simulink model "ProgramCounter"  (R2024b)
settings: Solver=FixedStepAuto  StartTime=0.0  StopTime=10  FixedStep=1e-6  RelTol=1e-3
libraries: simulink_extras x13
settings Model: PacingRate=0.002500  Creator=Erys  LastModifiedBy=Erys
settings SolverCC: AllowMultiTaskInputOutput=on

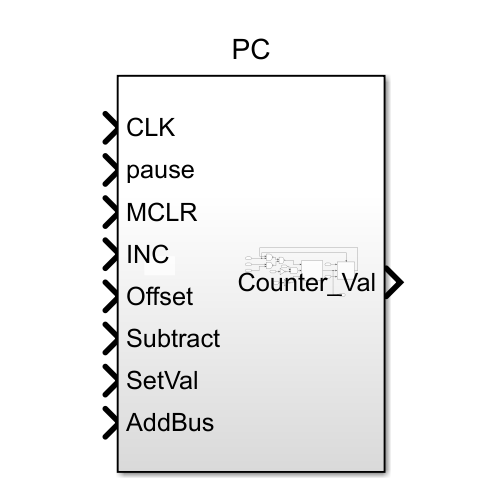
[thumbnail: Simulink's stored preview of the top-level diagram]
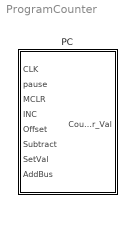
== system ProgramCounter ==
  PC : Subsystem

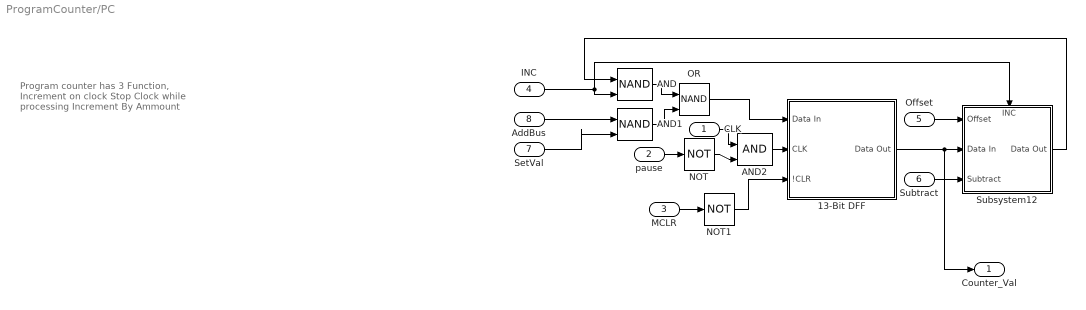
== system ProgramCounter/PC ==
  note: Program counter has 3 Function,
      |
      | Increment on clock
      | Stop Clock while processing
      | Increment By Ammount
  CLK : Inport
  pause : Inport  Port=2
  MCLR : Inport  Port=3
  INC : Inport  Port=4
  Offset : Inport  Port=5
  Subtract : Inport  Port=6
  SetVal : Inport  Port=7
  AddBus : Inport  Port=8
  "13-Bit DFF " : Subsystem
  AND : Logic  Operator=NAND  IconShape=distinctive  AllPortsSameDT=off  OutDataTypeStr=boolean
  AND1 : Logic  Operator=NAND  IconShape=distinctive  AllPortsSameDT=off  OutDataTypeStr=boolean
  AND2 : Logic  IconShape=distinctive  AllPortsSameDT=off  OutDataTypeStr=boolean
  NOT : Logic  Operator=NOT  IconShape=distinctive  AllPortsSameDT=off  OutDataTypeStr=boolean
  NOT1 : Logic  Operator=NOT  IconShape=distinctive  AllPortsSameDT=off  OutDataTypeStr=boolean
  OR : Logic  Operator=NAND  IconShape=distinctive  AllPortsSameDT=off  OutDataTypeStr=boolean
  Subsystem12 : Subsystem
      settings: PortSchema="{\"entries\":[{\"content\":{\"sides\":[{\"content\":{\"connectorIds\":[\"In1\",\"In2\",\"In3\"]},\"type\":\"ConnectorPlacement.EquallySpacedRectSide\",\"uuid\":\"739cec16-4094-4955-9615-f23c4a15ab23\"},{\"content\":{\"connectorIds\":[\"Out1\"],\"side\":\"RIGHT\"},\"type\":\"ConnectorPlacement.EquallySpacedRectSide\",\"uuid\":\"36202d39-d5af-435f-89aa-f53363edb9fe\"},{\"content\":{\"connectorIds\":[\"In4\"],\"side\":\"TOP\"},\"type\":\"ConnectorPlacement.EquallySpacedRectSide\",\"uuid\":\"08216fe9-0399-4cf5-9d97-18b54c3decd6\"}]},\"type\":\"ConnectorPlacement.EquallySpacedConnector\",\"uuid\":\"ce037f61-d800-42dc-bcb7-acda0bd23fde\"}],\"packageUris\":[\"http://schema.mathworks.com/mf0/Connector/R2020b\"],\"version\":\"1.0\"}"
  Counter_Val : Outport
  wires:
  CLK/1 -> AND2/1
  MCLR/1 -> NOT1/1
  "13-Bit DFF "/1(Data Out) -> Counter_Val/1, Subsystem12/2(Data In)
  Subsystem12/1(Data Out) -> AND/1
  AND/1 -> OR/1
  AND1/1 -> OR/2
  OR/1 -> "13-Bit DFF "/1(Data In)
  Offset/1 -> Subsystem12/1(Offset)
  INC/1 -> AND/2, Subsystem12/4(INC)
  Subtract/1 -> Subsystem12/3(Subtract)
  SetVal/1 -> AND1/2
  AddBus/1 -> AND1/1
  NOT/1 -> AND2/2
  pause/1 -> NOT/1
  NOT1/1 -> "13-Bit DFF "/3(!CLR)
  AND2/1 -> "13-Bit DFF "/2(CLK)

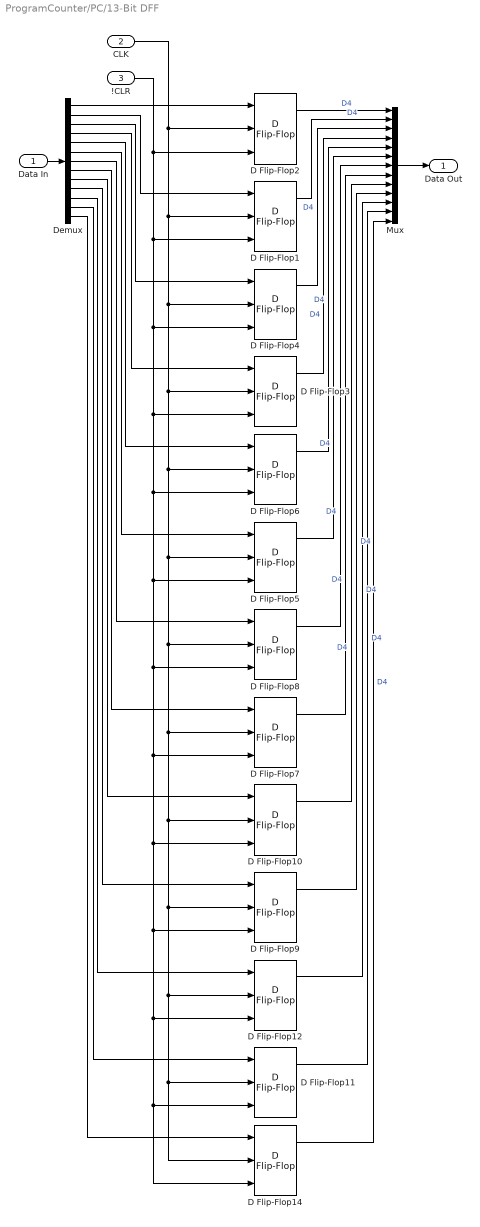
== system ProgramCounter/PC/13-Bit DFF  ==
  Data In : Inport
  CLK : Inport  Port=2
  !CLR : Inport  Port=3
  D Flip-Flop{1..12,14} (13 alike) : simulink_extras/Flip Flops/D Flip-Flop
  Demux : Demux  Outputs=13
  Mux : Mux  Inputs=13
  Data Out : Outport
  wires:
  Data In/1 -> Demux/1
  Mux/1 -> Data Out/1
  !CLR/1 -> D Flip-Flop4/3, D Flip-Flop3/3, D Flip-Flop6/3, D Flip-Flop8/3, D Flip-Flop12/3, D Flip-Flop11/3, D Flip-Flop14/3, D Flip-Flop9/3, D Flip-Flop10/3, D Flip-Flop7/3, D Flip-Flop5/3, D Flip-Flop1/3, D Flip-Flop2/3
  CLK/1 -> D Flip-Flop1/2, D Flip-Flop6/2, D Flip-Flop5/2, D Flip-Flop8/2, D Flip-Flop9/2, D Flip-Flop14/2, D Flip-Flop11/2, D Flip-Flop12/2, D Flip-Flop10/2, D Flip-Flop7/2, D Flip-Flop3/2, D Flip-Flop4/2, D Flip-Flop2/2
  Demux/1 -> D Flip-Flop2/1
  Demux/2 -> D Flip-Flop1/1
  Demux/3 -> D Flip-Flop4/1
  Demux/4 -> D Flip-Flop3/1
  Demux/5 -> D Flip-Flop6/1
  Demux/6 -> D Flip-Flop5/1
  Demux/7 -> D Flip-Flop8/1
  Demux/8 -> D Flip-Flop7/1
  Demux/9 -> D Flip-Flop10/1
  Demux/10 -> D Flip-Flop9/1
  Demux/11 -> D Flip-Flop12/1
  Demux/12 -> D Flip-Flop11/1
  Demux/13 -> D Flip-Flop14/1
  D Flip-Flop2/1 -> Mux/1  "D4"
  D Flip-Flop1/1 -> Mux/2  "D4"
  D Flip-Flop4/1 -> Mux/3  "D4"
  D Flip-Flop3/1 -> Mux/4  "D4"
  D Flip-Flop6/1 -> Mux/5  "D4"
  D Flip-Flop5/1 -> Mux/6  "D4"
  D Flip-Flop8/1 -> Mux/7  "D4"
  D Flip-Flop7/1 -> Mux/8  "D4"
  D Flip-Flop10/1 -> Mux/9  "D4"
  D Flip-Flop9/1 -> Mux/10  "D4"
  D Flip-Flop12/1 -> Mux/11  "D4"
  D Flip-Flop11/1 -> Mux/12  "D4"
  D Flip-Flop14/1 -> Mux/13  "D4"

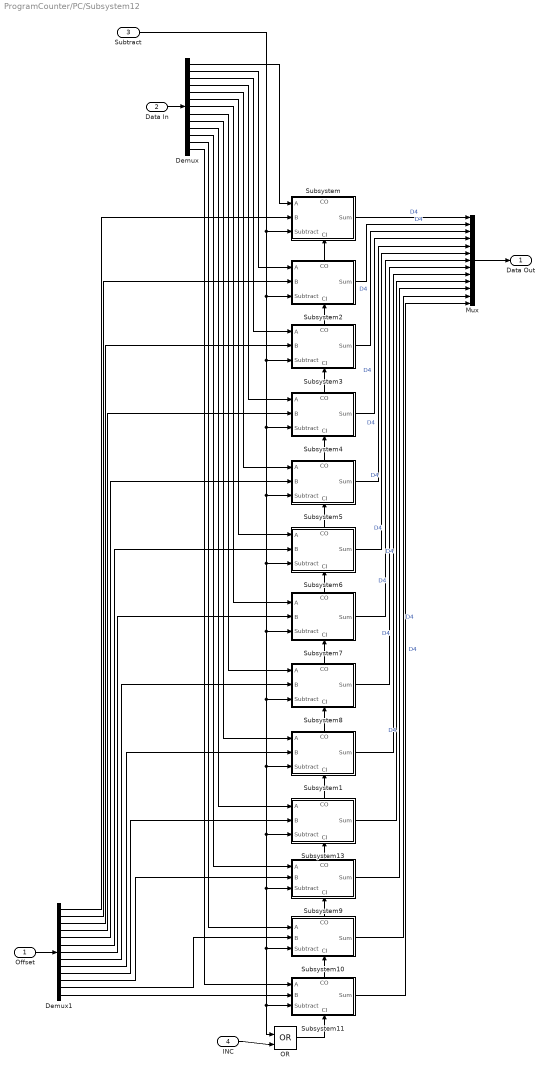
== system ProgramCounter/PC/Subsystem12 ==
  Offset : Inport
  Data In : Inport  Port=2
  Subtract : Inport  Port=3
  INC : Inport  Port=4
  Demux : Demux  Outputs=13
  Demux1 : Demux  Outputs=13
  Mux : Mux  Inputs=13
  OR : Logic  Operator=OR  IconShape=distinctive  AllPortsSameDT=off  OutDataTypeStr=boolean
  Subsystem : Subsystem
      settings: PortSchema="{\"entries\":[{\"content\":{\"sides\":[{\"content\":{\"connectorIds\":[\"In1\",\"In2\",\"In3\"]},\"type\":\"ConnectorPlacement.EquallySpacedRectSide\",\"uuid\":\"3b61df12-5278-441c-99ea-cd13bbe6a5f0\"},{\"content\":{\"connectorIds\":[\"Out1\"],\"side\":\"RIGHT\"},\"type\":\"ConnectorPlacement.EquallySpacedRectSide\",\"uuid\":\"d74b7cc5-7b27-4e0f-8d84-952eb44d2cfa\"},{\"content\":{\"connectorIds\":[\"Out2\"],\"side\":\"TOP\"},\"type\":\"ConnectorPlacement.EquallySpacedRectSide\",\"uuid\":\"99314f25-b6d9-4ea5-a032-83307ae4bc34\"},{\"content\":{\"connectorIds\":[\"In4\"],\"side\":\"BOTTOM\"},\"type\":\"ConnectorPlacement.EquallySpacedRectSide\",\"uuid\":\"c9c43d88-8d1b-4564-af22-30722c8258ba\"}]},\"type\":\"ConnectorPlacement.EquallySpacedConnector\",\"uuid\":\"25cc7102-d96a-4215-b1b2-f44cf7e448cb\"}],\"packageUris\":[\"http://schema.mathworks.com/mf0/Connector/R2020b\"],\"version\":\"1.0\"}"
  Subsystem1 : Subsystem
      settings: PortSchema="{\"entries\":[{\"content\":{\"sides\":[{\"content\":{\"connectorIds\":[\"In1\",\"In2\",\"In3\"]},\"type\":\"ConnectorPlacement.EquallySpacedRectSide\",\"uuid\":\"3b61df12-5278-441c-99ea-cd13bbe6a5f0\"},{\"content\":{\"connectorIds\":[\"Out1\"],\"side\":\"RIGHT\"},\"type\":\"ConnectorPlacement.EquallySpacedRectSide\",\"uuid\":\"d74b7cc5-7b27-4e0f-8d84-952eb44d2cfa\"},{\"content\":{\"connectorIds\":[\"Out2\"],\"side\":\"TOP\"},\"type\":\"ConnectorPlacement.EquallySpacedRectSide\",\"uuid\":\"99314f25-b6d9-4ea5-a032-83307ae4bc34\"},{\"content\":{\"connectorIds\":[\"In4\"],\"side\":\"BOTTOM\"},\"type\":\"ConnectorPlacement.EquallySpacedRectSide\",\"uuid\":\"c9c43d88-8d1b-4564-af22-30722c8258ba\"}]},\"type\":\"ConnectorPlacement.EquallySpacedConnector\",\"uuid\":\"25cc7102-d96a-4215-b1b2-f44cf7e448cb\"}],\"packageUris\":[\"http://schema.mathworks.com/mf0/Connector/R2020b\"],\"version\":\"1.0\"}"
  Subsystem10 : Subsystem
      settings: PortSchema="{\"entries\":[{\"content\":{\"sides\":[{\"content\":{\"connectorIds\":[\"In1\",\"In2\",\"In3\"]},\"type\":\"ConnectorPlacement.EquallySpacedRectSide\",\"uuid\":\"3b61df12-5278-441c-99ea-cd13bbe6a5f0\"},{\"content\":{\"connectorIds\":[\"Out1\"],\"side\":\"RIGHT\"},\"type\":\"ConnectorPlacement.EquallySpacedRectSide\",\"uuid\":\"d74b7cc5-7b27-4e0f-8d84-952eb44d2cfa\"},{\"content\":{\"connectorIds\":[\"Out2\"],\"side\":\"TOP\"},\"type\":\"ConnectorPlacement.EquallySpacedRectSide\",\"uuid\":\"99314f25-b6d9-4ea5-a032-83307ae4bc34\"},{\"content\":{\"connectorIds\":[\"In4\"],\"side\":\"BOTTOM\"},\"type\":\"ConnectorPlacement.EquallySpacedRectSide\",\"uuid\":\"c9c43d88-8d1b-4564-af22-30722c8258ba\"}]},\"type\":\"ConnectorPlacement.EquallySpacedConnector\",\"uuid\":\"25cc7102-d96a-4215-b1b2-f44cf7e448cb\"}],\"packageUris\":[\"http://schema.mathworks.com/mf0/Connector/R2020b\"],\"version\":\"1.0\"}"
  Subsystem11 : Subsystem
      settings: PortSchema="{\"entries\":[{\"content\":{\"sides\":[{\"content\":{\"connectorIds\":[\"In1\",\"In2\",\"In3\"]},\"type\":\"ConnectorPlacement.EquallySpacedRectSide\",\"uuid\":\"3b61df12-5278-441c-99ea-cd13bbe6a5f0\"},{\"content\":{\"connectorIds\":[\"Out1\"],\"side\":\"RIGHT\"},\"type\":\"ConnectorPlacement.EquallySpacedRectSide\",\"uuid\":\"d74b7cc5-7b27-4e0f-8d84-952eb44d2cfa\"},{\"content\":{\"connectorIds\":[\"Out2\"],\"side\":\"TOP\"},\"type\":\"ConnectorPlacement.EquallySpacedRectSide\",\"uuid\":\"99314f25-b6d9-4ea5-a032-83307ae4bc34\"},{\"content\":{\"connectorIds\":[\"In4\"],\"side\":\"BOTTOM\"},\"type\":\"ConnectorPlacement.EquallySpacedRectSide\",\"uuid\":\"c9c43d88-8d1b-4564-af22-30722c8258ba\"}]},\"type\":\"ConnectorPlacement.EquallySpacedConnector\",\"uuid\":\"25cc7102-d96a-4215-b1b2-f44cf7e448cb\"}],\"packageUris\":[\"http://schema.mathworks.com/mf0/Connector/R2020b\"],\"version\":\"1.0\"}"
  Subsystem13 : Subsystem
      settings: PortSchema="{\"entries\":[{\"content\":{\"sides\":[{\"content\":{\"connectorIds\":[\"In1\",\"In2\",\"In3\"]},\"type\":\"ConnectorPlacement.EquallySpacedRectSide\",\"uuid\":\"3b61df12-5278-441c-99ea-cd13bbe6a5f0\"},{\"content\":{\"connectorIds\":[\"Out1\"],\"side\":\"RIGHT\"},\"type\":\"ConnectorPlacement.EquallySpacedRectSide\",\"uuid\":\"d74b7cc5-7b27-4e0f-8d84-952eb44d2cfa\"},{\"content\":{\"connectorIds\":[\"Out2\"],\"side\":\"TOP\"},\"type\":\"ConnectorPlacement.EquallySpacedRectSide\",\"uuid\":\"99314f25-b6d9-4ea5-a032-83307ae4bc34\"},{\"content\":{\"connectorIds\":[\"In4\"],\"side\":\"BOTTOM\"},\"type\":\"ConnectorPlacement.EquallySpacedRectSide\",\"uuid\":\"c9c43d88-8d1b-4564-af22-30722c8258ba\"}]},\"type\":\"ConnectorPlacement.EquallySpacedConnector\",\"uuid\":\"25cc7102-d96a-4215-b1b2-f44cf7e448cb\"}],\"packageUris\":[\"http://schema.mathworks.com/mf0/Connector/R2020b\"],\"version\":\"1.0\"}"
  Subsystem2 : Subsystem
      settings: PortSchema="{\"entries\":[{\"content\":{\"sides\":[{\"content\":{\"connectorIds\":[\"In1\",\"In2\",\"In3\"]},\"type\":\"ConnectorPlacement.EquallySpacedRectSide\",\"uuid\":\"3b61df12-5278-441c-99ea-cd13bbe6a5f0\"},{\"content\":{\"connectorIds\":[\"Out1\"],\"side\":\"RIGHT\"},\"type\":\"ConnectorPlacement.EquallySpacedRectSide\",\"uuid\":\"d74b7cc5-7b27-4e0f-8d84-952eb44d2cfa\"},{\"content\":{\"connectorIds\":[\"Out2\"],\"side\":\"TOP\"},\"type\":\"ConnectorPlacement.EquallySpacedRectSide\",\"uuid\":\"99314f25-b6d9-4ea5-a032-83307ae4bc34\"},{\"content\":{\"connectorIds\":[\"In4\"],\"side\":\"BOTTOM\"},\"type\":\"ConnectorPlacement.EquallySpacedRectSide\",\"uuid\":\"c9c43d88-8d1b-4564-af22-30722c8258ba\"}]},\"type\":\"ConnectorPlacement.EquallySpacedConnector\",\"uuid\":\"25cc7102-d96a-4215-b1b2-f44cf7e448cb\"}],\"packageUris\":[\"http://schema.mathworks.com/mf0/Connector/R2020b\"],\"version\":\"1.0\"}"
  Subsystem3 : Subsystem
      settings: PortSchema="{\"entries\":[{\"content\":{\"sides\":[{\"content\":{\"connectorIds\":[\"In1\",\"In2\",\"In3\"]},\"type\":\"ConnectorPlacement.EquallySpacedRectSide\",\"uuid\":\"3b61df12-5278-441c-99ea-cd13bbe6a5f0\"},{\"content\":{\"connectorIds\":[\"Out1\"],\"side\":\"RIGHT\"},\"type\":\"ConnectorPlacement.EquallySpacedRectSide\",\"uuid\":\"d74b7cc5-7b27-4e0f-8d84-952eb44d2cfa\"},{\"content\":{\"connectorIds\":[\"Out2\"],\"side\":\"TOP\"},\"type\":\"ConnectorPlacement.EquallySpacedRectSide\",\"uuid\":\"99314f25-b6d9-4ea5-a032-83307ae4bc34\"},{\"content\":{\"connectorIds\":[\"In4\"],\"side\":\"BOTTOM\"},\"type\":\"ConnectorPlacement.EquallySpacedRectSide\",\"uuid\":\"c9c43d88-8d1b-4564-af22-30722c8258ba\"}]},\"type\":\"ConnectorPlacement.EquallySpacedConnector\",\"uuid\":\"25cc7102-d96a-4215-b1b2-f44cf7e448cb\"}],\"packageUris\":[\"http://schema.mathworks.com/mf0/Connector/R2020b\"],\"version\":\"1.0\"}"
  Subsystem4 : Subsystem
      settings: PortSchema="{\"entries\":[{\"content\":{\"sides\":[{\"content\":{\"connectorIds\":[\"In1\",\"In2\",\"In3\"]},\"type\":\"ConnectorPlacement.EquallySpacedRectSide\",\"uuid\":\"3b61df12-5278-441c-99ea-cd13bbe6a5f0\"},{\"content\":{\"connectorIds\":[\"Out1\"],\"side\":\"RIGHT\"},\"type\":\"ConnectorPlacement.EquallySpacedRectSide\",\"uuid\":\"d74b7cc5-7b27-4e0f-8d84-952eb44d2cfa\"},{\"content\":{\"connectorIds\":[\"Out2\"],\"side\":\"TOP\"},\"type\":\"ConnectorPlacement.EquallySpacedRectSide\",\"uuid\":\"99314f25-b6d9-4ea5-a032-83307ae4bc34\"},{\"content\":{\"connectorIds\":[\"In4\"],\"side\":\"BOTTOM\"},\"type\":\"ConnectorPlacement.EquallySpacedRectSide\",\"uuid\":\"c9c43d88-8d1b-4564-af22-30722c8258ba\"}]},\"type\":\"ConnectorPlacement.EquallySpacedConnector\",\"uuid\":\"25cc7102-d96a-4215-b1b2-f44cf7e448cb\"}],\"packageUris\":[\"http://schema.mathworks.com/mf0/Connector/R2020b\"],\"version\":\"1.0\"}"
  Subsystem5 : Subsystem
      settings: PortSchema="{\"entries\":[{\"content\":{\"sides\":[{\"content\":{\"connectorIds\":[\"In1\",\"In2\",\"In3\"]},\"type\":\"ConnectorPlacement.EquallySpacedRectSide\",\"uuid\":\"3b61df12-5278-441c-99ea-cd13bbe6a5f0\"},{\"content\":{\"connectorIds\":[\"Out1\"],\"side\":\"RIGHT\"},\"type\":\"ConnectorPlacement.EquallySpacedRectSide\",\"uuid\":\"d74b7cc5-7b27-4e0f-8d84-952eb44d2cfa\"},{\"content\":{\"connectorIds\":[\"Out2\"],\"side\":\"TOP\"},\"type\":\"ConnectorPlacement.EquallySpacedRectSide\",\"uuid\":\"99314f25-b6d9-4ea5-a032-83307ae4bc34\"},{\"content\":{\"connectorIds\":[\"In4\"],\"side\":\"BOTTOM\"},\"type\":\"ConnectorPlacement.EquallySpacedRectSide\",\"uuid\":\"c9c43d88-8d1b-4564-af22-30722c8258ba\"}]},\"type\":\"ConnectorPlacement.EquallySpacedConnector\",\"uuid\":\"25cc7102-d96a-4215-b1b2-f44cf7e448cb\"}],\"packageUris\":[\"http://schema.mathworks.com/mf0/Connector/R2020b\"],\"version\":\"1.0\"}"
  Subsystem6 : Subsystem
      settings: PortSchema="{\"entries\":[{\"content\":{\"sides\":[{\"content\":{\"connectorIds\":[\"In1\",\"In2\",\"In3\"]},\"type\":\"ConnectorPlacement.EquallySpacedRectSide\",\"uuid\":\"3b61df12-5278-441c-99ea-cd13bbe6a5f0\"},{\"content\":{\"connectorIds\":[\"Out1\"],\"side\":\"RIGHT\"},\"type\":\"ConnectorPlacement.EquallySpacedRectSide\",\"uuid\":\"d74b7cc5-7b27-4e0f-8d84-952eb44d2cfa\"},{\"content\":{\"connectorIds\":[\"Out2\"],\"side\":\"TOP\"},\"type\":\"ConnectorPlacement.EquallySpacedRectSide\",\"uuid\":\"99314f25-b6d9-4ea5-a032-83307ae4bc34\"},{\"content\":{\"connectorIds\":[\"In4\"],\"side\":\"BOTTOM\"},\"type\":\"ConnectorPlacement.EquallySpacedRectSide\",\"uuid\":\"c9c43d88-8d1b-4564-af22-30722c8258ba\"}]},\"type\":\"ConnectorPlacement.EquallySpacedConnector\",\"uuid\":\"25cc7102-d96a-4215-b1b2-f44cf7e448cb\"}],\"packageUris\":[\"http://schema.mathworks.com/mf0/Connector/R2020b\"],\"version\":\"1.0\"}"
  Subsystem7 : Subsystem
      settings: PortSchema="{\"entries\":[{\"content\":{\"sides\":[{\"content\":{\"connectorIds\":[\"In1\",\"In2\",\"In3\"]},\"type\":\"ConnectorPlacement.EquallySpacedRectSide\",\"uuid\":\"3b61df12-5278-441c-99ea-cd13bbe6a5f0\"},{\"content\":{\"connectorIds\":[\"Out1\"],\"side\":\"RIGHT\"},\"type\":\"ConnectorPlacement.EquallySpacedRectSide\",\"uuid\":\"d74b7cc5-7b27-4e0f-8d84-952eb44d2cfa\"},{\"content\":{\"connectorIds\":[\"Out2\"],\"side\":\"TOP\"},\"type\":\"ConnectorPlacement.EquallySpacedRectSide\",\"uuid\":\"99314f25-b6d9-4ea5-a032-83307ae4bc34\"},{\"content\":{\"connectorIds\":[\"In4\"],\"side\":\"BOTTOM\"},\"type\":\"ConnectorPlacement.EquallySpacedRectSide\",\"uuid\":\"c9c43d88-8d1b-4564-af22-30722c8258ba\"}]},\"type\":\"ConnectorPlacement.EquallySpacedConnector\",\"uuid\":\"25cc7102-d96a-4215-b1b2-f44cf7e448cb\"}],\"packageUris\":[\"http://schema.mathworks.com/mf0/Connector/R2020b\"],\"version\":\"1.0\"}"
  Subsystem8 : Subsystem
      settings: PortSchema="{\"entries\":[{\"content\":{\"sides\":[{\"content\":{\"connectorIds\":[\"In1\",\"In2\",\"In3\"]},\"type\":\"ConnectorPlacement.EquallySpacedRectSide\",\"uuid\":\"3b61df12-5278-441c-99ea-cd13bbe6a5f0\"},{\"content\":{\"connectorIds\":[\"Out1\"],\"side\":\"RIGHT\"},\"type\":\"ConnectorPlacement.EquallySpacedRectSide\",\"uuid\":\"d74b7cc5-7b27-4e0f-8d84-952eb44d2cfa\"},{\"content\":{\"connectorIds\":[\"Out2\"],\"side\":\"TOP\"},\"type\":\"ConnectorPlacement.EquallySpacedRectSide\",\"uuid\":\"99314f25-b6d9-4ea5-a032-83307ae4bc34\"},{\"content\":{\"connectorIds\":[\"In4\"],\"side\":\"BOTTOM\"},\"type\":\"ConnectorPlacement.EquallySpacedRectSide\",\"uuid\":\"c9c43d88-8d1b-4564-af22-30722c8258ba\"}]},\"type\":\"ConnectorPlacement.EquallySpacedConnector\",\"uuid\":\"25cc7102-d96a-4215-b1b2-f44cf7e448cb\"}],\"packageUris\":[\"http://schema.mathworks.com/mf0/Connector/R2020b\"],\"version\":\"1.0\"}"
  Subsystem9 : Subsystem
      settings: PortSchema="{\"entries\":[{\"content\":{\"sides\":[{\"content\":{\"connectorIds\":[\"In1\",\"In2\",\"In3\"]},\"type\":\"ConnectorPlacement.EquallySpacedRectSide\",\"uuid\":\"3b61df12-5278-441c-99ea-cd13bbe6a5f0\"},{\"content\":{\"connectorIds\":[\"Out1\"],\"side\":\"RIGHT\"},\"type\":\"ConnectorPlacement.EquallySpacedRectSide\",\"uuid\":\"d74b7cc5-7b27-4e0f-8d84-952eb44d2cfa\"},{\"content\":{\"connectorIds\":[\"Out2\"],\"side\":\"TOP\"},\"type\":\"ConnectorPlacement.EquallySpacedRectSide\",\"uuid\":\"99314f25-b6d9-4ea5-a032-83307ae4bc34\"},{\"content\":{\"connectorIds\":[\"In4\"],\"side\":\"BOTTOM\"},\"type\":\"ConnectorPlacement.EquallySpacedRectSide\",\"uuid\":\"c9c43d88-8d1b-4564-af22-30722c8258ba\"}]},\"type\":\"ConnectorPlacement.EquallySpacedConnector\",\"uuid\":\"25cc7102-d96a-4215-b1b2-f44cf7e448cb\"}],\"packageUris\":[\"http://schema.mathworks.com/mf0/Connector/R2020b\"],\"version\":\"1.0\"}"
  Data Out : Outport
  wires:
  Demux/2 -> Subsystem2/1(A)
  Subtract/1 -> Subsystem/3(Subtract), OR/1, Subsystem11/3(Subtract), Subsystem10/3(Subtract), Subsystem9/3(Subtract), Subsystem13/3(Subtract), Subsystem1/3(Subtract), Subsystem8/3(Subtract), Subsystem7/3(Subtract), Subsystem6/3(Subtract), Subsystem5/3(Subtract), Subsystem4/3(Subtract), Subsystem3/3(Subtract), Subsystem2/3(Subtract)
  Subsystem8/2(CO) -> Subsystem7/4(CI)
  Demux/10 -> Subsystem13/1(A)
  Subsystem10/2(CO) -> Subsystem9/4(CI)
  Demux/1 -> Subsystem/1(A)
  Subsystem11/2(CO) -> Subsystem10/4(CI)
  Demux/5 -> Subsystem5/1(A)
  Subsystem10/1(Sum) -> Mux/12  "D4"
  Demux/7 -> Subsystem7/1(A)
  Subsystem3/1(Sum) -> Mux/3  "D4"
  Subsystem6/1(Sum) -> Mux/6  "D4"
  Demux/13 -> Subsystem11/1(A)
  Subsystem5/2(CO) -> Subsystem4/4(CI)
  Demux1/11 -> Subsystem9/2(B)
  OR/1 -> Subsystem11/4(CI)
  Demux1/12 -> Subsystem10/2(B)
  Offset/1 -> Demux1/1
  Subsystem2/1(Sum) -> Mux/2  "D4"
  Demux1/9 -> Subsystem1/2(B)
  INC/1 -> OR/2
  Demux1/13 -> Subsystem11/2(B)
  Demux1/8 -> Subsystem8/2(B)
  Demux1/10 -> Subsystem13/2(B)
  Demux1/2 -> Subsystem2/2(B)
  Demux1/1 -> Subsystem/2(B)
  Demux1/6 -> Subsystem6/2(B)
  Subsystem/1(Sum) -> Mux/1  "D4"
  Demux1/3 -> Subsystem3/2(B)
  Demux1/7 -> Subsystem7/2(B)
  Demux1/4 -> Subsystem4/2(B)
  Subsystem4/2(CO) -> Subsystem3/4(CI)
  Subsystem7/1(Sum) -> Mux/7  "D4"
  Demux/6 -> Subsystem6/1(A)
  Subsystem6/2(CO) -> Subsystem5/4(CI)
  Demux1/5 -> Subsystem5/2(B)
  Subsystem7/2(CO) -> Subsystem6/4(CI)
  Subsystem3/2(CO) -> Subsystem2/4(CI)
  Subsystem5/1(Sum) -> Mux/5  "D4"
  Subsystem2/2(CO) -> Subsystem/4(CI)
  Subsystem1/1(Sum) -> Mux/9  "D4"
  Subsystem8/1(Sum) -> Mux/8  "D4"
  Subsystem11/1(Sum) -> Mux/13  "D4"
  Subsystem13/2(CO) -> Subsystem1/4(CI)
  Subsystem9/1(Sum) -> Mux/11  "D4"
  Subsystem1/2(CO) -> Subsystem8/4(CI)
  Demux/9 -> Subsystem1/1(A)
  Demux/11 -> Subsystem9/1(A)
  Mux/1 -> Data Out/1
  Subsystem9/2(CO) -> Subsystem13/4(CI)
  Subsystem13/1(Sum) -> Mux/10  "D4"
  Demux/8 -> Subsystem8/1(A)
  Demux/4 -> Subsystem4/1(A)
  Data In/1 -> Demux/1
  Subsystem4/1(Sum) -> Mux/4  "D4"
  Demux/3 -> Subsystem3/1(A)
  Demux/12 -> Subsystem10/1(A)

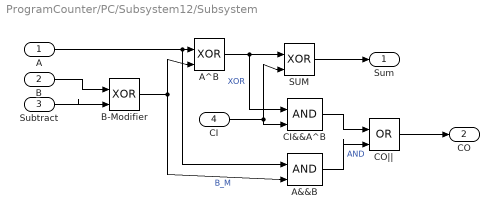
== system ProgramCounter/PC/Subsystem12/Subsystem ==
  A : Inport
  B : Inport  Port=2
  Subtract : Inport  Port=3
  CI : Inport  Port=4
  A&&B : Logic  IconShape=distinctive  AllPortsSameDT=off  OutDataTypeStr=boolean
  A^B : Logic  Operator=XOR  IconShape=distinctive  AllPortsSameDT=off  OutDataTypeStr=boolean
  B-Modifier : Logic  Operator=XOR  IconShape=distinctive  AllPortsSameDT=off  OutDataTypeStr=boolean
  CI&&A^B : Logic  IconShape=distinctive  AllPortsSameDT=off  OutDataTypeStr=boolean
  CO|| : Logic  Operator=OR  IconShape=distinctive  AllPortsSameDT=off  OutDataTypeStr=boolean
  SUM : Logic  Operator=XOR  IconShape=distinctive  AllPortsSameDT=off  OutDataTypeStr=boolean
  Sum : Outport
  CO : Outport  Port=2
  wires:
  B/1 -> B-Modifier/1
  Subtract/1 -> B-Modifier/2
  CI&&A^B/1 -> CO||/1
  A&&B/1 -> CO||/2  "AND"
  CO||/1 -> CO/1
  B-Modifier/1 -> A&&B/2, A^B/2  "B_M"
  CI/1 -> CI&&A^B/2, SUM/2
  A^B/1 -> CI&&A^B/1, SUM/1  "XOR"
  A/1 -> A&&B/1, A^B/1
  SUM/1 -> Sum/1

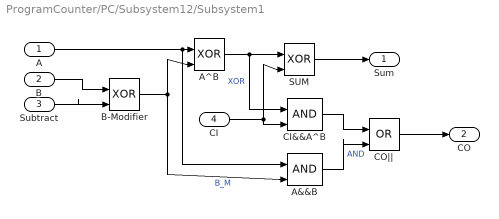
== system ProgramCounter/PC/Subsystem12/Subsystem1 ==
  A : Inport
  B : Inport  Port=2
  Subtract : Inport  Port=3
  CI : Inport  Port=4
  A&&B : Logic  IconShape=distinctive  AllPortsSameDT=off  OutDataTypeStr=boolean
  A^B : Logic  Operator=XOR  IconShape=distinctive  AllPortsSameDT=off  OutDataTypeStr=boolean
  B-Modifier : Logic  Operator=XOR  IconShape=distinctive  AllPortsSameDT=off  OutDataTypeStr=boolean
  CI&&A^B : Logic  IconShape=distinctive  AllPortsSameDT=off  OutDataTypeStr=boolean
  CO|| : Logic  Operator=OR  IconShape=distinctive  AllPortsSameDT=off  OutDataTypeStr=boolean
  SUM : Logic  Operator=XOR  IconShape=distinctive  AllPortsSameDT=off  OutDataTypeStr=boolean
  Sum : Outport
  CO : Outport  Port=2
  wires:
  B/1 -> B-Modifier/1
  Subtract/1 -> B-Modifier/2
  CI&&A^B/1 -> CO||/1
  A&&B/1 -> CO||/2  "AND"
  CO||/1 -> CO/1
  B-Modifier/1 -> A&&B/2, A^B/2  "B_M"
  CI/1 -> CI&&A^B/2, SUM/2
  A^B/1 -> CI&&A^B/1, SUM/1  "XOR"
  A/1 -> A&&B/1, A^B/1
  SUM/1 -> Sum/1

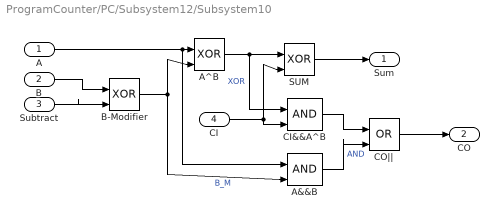
== system ProgramCounter/PC/Subsystem12/Subsystem10 ==
  A : Inport
  B : Inport  Port=2
  Subtract : Inport  Port=3
  CI : Inport  Port=4
  A&&B : Logic  IconShape=distinctive  AllPortsSameDT=off  OutDataTypeStr=boolean
  A^B : Logic  Operator=XOR  IconShape=distinctive  AllPortsSameDT=off  OutDataTypeStr=boolean
  B-Modifier : Logic  Operator=XOR  IconShape=distinctive  AllPortsSameDT=off  OutDataTypeStr=boolean
  CI&&A^B : Logic  IconShape=distinctive  AllPortsSameDT=off  OutDataTypeStr=boolean
  CO|| : Logic  Operator=OR  IconShape=distinctive  AllPortsSameDT=off  OutDataTypeStr=boolean
  SUM : Logic  Operator=XOR  IconShape=distinctive  AllPortsSameDT=off  OutDataTypeStr=boolean
  Sum : Outport
  CO : Outport  Port=2
  wires:
  B/1 -> B-Modifier/1
  Subtract/1 -> B-Modifier/2
  CI&&A^B/1 -> CO||/1
  A&&B/1 -> CO||/2  "AND"
  CO||/1 -> CO/1
  B-Modifier/1 -> A&&B/2, A^B/2  "B_M"
  CI/1 -> CI&&A^B/2, SUM/2
  A^B/1 -> CI&&A^B/1, SUM/1  "XOR"
  A/1 -> A&&B/1, A^B/1
  SUM/1 -> Sum/1

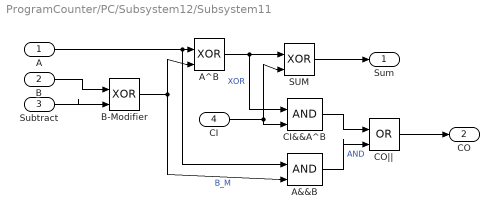
== system ProgramCounter/PC/Subsystem12/Subsystem11 ==
  A : Inport
  B : Inport  Port=2
  Subtract : Inport  Port=3
  CI : Inport  Port=4
  A&&B : Logic  IconShape=distinctive  AllPortsSameDT=off  OutDataTypeStr=boolean
  A^B : Logic  Operator=XOR  IconShape=distinctive  AllPortsSameDT=off  OutDataTypeStr=boolean
  B-Modifier : Logic  Operator=XOR  IconShape=distinctive  AllPortsSameDT=off  OutDataTypeStr=boolean
  CI&&A^B : Logic  IconShape=distinctive  AllPortsSameDT=off  OutDataTypeStr=boolean
  CO|| : Logic  Operator=OR  IconShape=distinctive  AllPortsSameDT=off  OutDataTypeStr=boolean
  SUM : Logic  Operator=XOR  IconShape=distinctive  AllPortsSameDT=off  OutDataTypeStr=boolean
  Sum : Outport
  CO : Outport  Port=2
  wires:
  B/1 -> B-Modifier/1
  Subtract/1 -> B-Modifier/2
  CI&&A^B/1 -> CO||/1
  A&&B/1 -> CO||/2  "AND"
  CO||/1 -> CO/1
  B-Modifier/1 -> A&&B/2, A^B/2  "B_M"
  CI/1 -> CI&&A^B/2, SUM/2
  A^B/1 -> CI&&A^B/1, SUM/1  "XOR"
  A/1 -> A&&B/1, A^B/1
  SUM/1 -> Sum/1

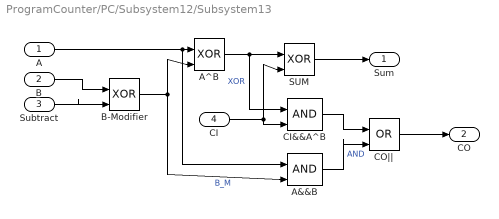
== system ProgramCounter/PC/Subsystem12/Subsystem13 ==
  A : Inport
  B : Inport  Port=2
  Subtract : Inport  Port=3
  CI : Inport  Port=4
  A&&B : Logic  IconShape=distinctive  AllPortsSameDT=off  OutDataTypeStr=boolean
  A^B : Logic  Operator=XOR  IconShape=distinctive  AllPortsSameDT=off  OutDataTypeStr=boolean
  B-Modifier : Logic  Operator=XOR  IconShape=distinctive  AllPortsSameDT=off  OutDataTypeStr=boolean
  CI&&A^B : Logic  IconShape=distinctive  AllPortsSameDT=off  OutDataTypeStr=boolean
  CO|| : Logic  Operator=OR  IconShape=distinctive  AllPortsSameDT=off  OutDataTypeStr=boolean
  SUM : Logic  Operator=XOR  IconShape=distinctive  AllPortsSameDT=off  OutDataTypeStr=boolean
  Sum : Outport
  CO : Outport  Port=2
  wires:
  B/1 -> B-Modifier/1
  Subtract/1 -> B-Modifier/2
  CI&&A^B/1 -> CO||/1
  A&&B/1 -> CO||/2  "AND"
  CO||/1 -> CO/1
  B-Modifier/1 -> A&&B/2, A^B/2  "B_M"
  CI/1 -> CI&&A^B/2, SUM/2
  A^B/1 -> CI&&A^B/1, SUM/1  "XOR"
  A/1 -> A&&B/1, A^B/1
  SUM/1 -> Sum/1

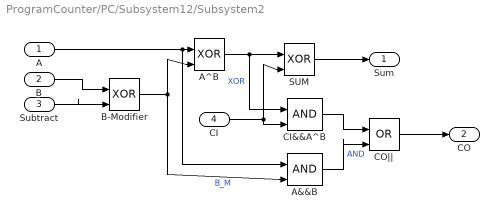
== system ProgramCounter/PC/Subsystem12/Subsystem2 ==
  A : Inport
  B : Inport  Port=2
  Subtract : Inport  Port=3
  CI : Inport  Port=4
  A&&B : Logic  IconShape=distinctive  AllPortsSameDT=off  OutDataTypeStr=boolean
  A^B : Logic  Operator=XOR  IconShape=distinctive  AllPortsSameDT=off  OutDataTypeStr=boolean
  B-Modifier : Logic  Operator=XOR  IconShape=distinctive  AllPortsSameDT=off  OutDataTypeStr=boolean
  CI&&A^B : Logic  IconShape=distinctive  AllPortsSameDT=off  OutDataTypeStr=boolean
  CO|| : Logic  Operator=OR  IconShape=distinctive  AllPortsSameDT=off  OutDataTypeStr=boolean
  SUM : Logic  Operator=XOR  IconShape=distinctive  AllPortsSameDT=off  OutDataTypeStr=boolean
  Sum : Outport
  CO : Outport  Port=2
  wires:
  B/1 -> B-Modifier/1
  Subtract/1 -> B-Modifier/2
  CI&&A^B/1 -> CO||/1
  A&&B/1 -> CO||/2  "AND"
  CO||/1 -> CO/1
  B-Modifier/1 -> A&&B/2, A^B/2  "B_M"
  CI/1 -> CI&&A^B/2, SUM/2
  A^B/1 -> CI&&A^B/1, SUM/1  "XOR"
  A/1 -> A&&B/1, A^B/1
  SUM/1 -> Sum/1

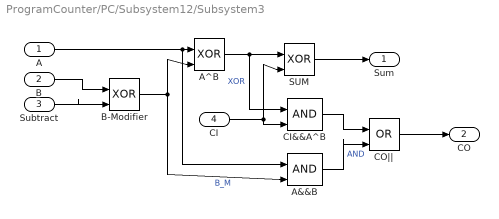
== system ProgramCounter/PC/Subsystem12/Subsystem3 ==
  A : Inport
  B : Inport  Port=2
  Subtract : Inport  Port=3
  CI : Inport  Port=4
  A&&B : Logic  IconShape=distinctive  AllPortsSameDT=off  OutDataTypeStr=boolean
  A^B : Logic  Operator=XOR  IconShape=distinctive  AllPortsSameDT=off  OutDataTypeStr=boolean
  B-Modifier : Logic  Operator=XOR  IconShape=distinctive  AllPortsSameDT=off  OutDataTypeStr=boolean
  CI&&A^B : Logic  IconShape=distinctive  AllPortsSameDT=off  OutDataTypeStr=boolean
  CO|| : Logic  Operator=OR  IconShape=distinctive  AllPortsSameDT=off  OutDataTypeStr=boolean
  SUM : Logic  Operator=XOR  IconShape=distinctive  AllPortsSameDT=off  OutDataTypeStr=boolean
  Sum : Outport
  CO : Outport  Port=2
  wires:
  B/1 -> B-Modifier/1
  Subtract/1 -> B-Modifier/2
  CI&&A^B/1 -> CO||/1
  A&&B/1 -> CO||/2  "AND"
  CO||/1 -> CO/1
  B-Modifier/1 -> A&&B/2, A^B/2  "B_M"
  CI/1 -> CI&&A^B/2, SUM/2
  A^B/1 -> CI&&A^B/1, SUM/1  "XOR"
  A/1 -> A&&B/1, A^B/1
  SUM/1 -> Sum/1

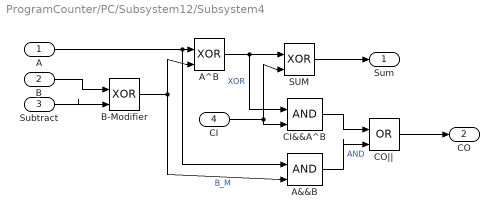
== system ProgramCounter/PC/Subsystem12/Subsystem4 ==
  A : Inport
  B : Inport  Port=2
  Subtract : Inport  Port=3
  CI : Inport  Port=4
  A&&B : Logic  IconShape=distinctive  AllPortsSameDT=off  OutDataTypeStr=boolean
  A^B : Logic  Operator=XOR  IconShape=distinctive  AllPortsSameDT=off  OutDataTypeStr=boolean
  B-Modifier : Logic  Operator=XOR  IconShape=distinctive  AllPortsSameDT=off  OutDataTypeStr=boolean
  CI&&A^B : Logic  IconShape=distinctive  AllPortsSameDT=off  OutDataTypeStr=boolean
  CO|| : Logic  Operator=OR  IconShape=distinctive  AllPortsSameDT=off  OutDataTypeStr=boolean
  SUM : Logic  Operator=XOR  IconShape=distinctive  AllPortsSameDT=off  OutDataTypeStr=boolean
  Sum : Outport
  CO : Outport  Port=2
  wires:
  B/1 -> B-Modifier/1
  Subtract/1 -> B-Modifier/2
  CI&&A^B/1 -> CO||/1
  A&&B/1 -> CO||/2  "AND"
  CO||/1 -> CO/1
  B-Modifier/1 -> A&&B/2, A^B/2  "B_M"
  CI/1 -> CI&&A^B/2, SUM/2
  A^B/1 -> CI&&A^B/1, SUM/1  "XOR"
  A/1 -> A&&B/1, A^B/1
  SUM/1 -> Sum/1

== system ProgramCounter/PC/Subsystem12/Subsystem5 ==
  A : Inport
  B : Inport  Port=2
  Subtract : Inport  Port=3
  CI : Inport  Port=4
  A&&B : Logic  IconShape=distinctive  AllPortsSameDT=off  OutDataTypeStr=boolean
  A^B : Logic  Operator=XOR  IconShape=distinctive  AllPortsSameDT=off  OutDataTypeStr=boolean
  B-Modifier : Logic  Operator=XOR  IconShape=distinctive  AllPortsSameDT=off  OutDataTypeStr=boolean
  CI&&A^B : Logic  IconShape=distinctive  AllPortsSameDT=off  OutDataTypeStr=boolean
  CO|| : Logic  Operator=OR  IconShape=distinctive  AllPortsSameDT=off  OutDataTypeStr=boolean
  SUM : Logic  Operator=XOR  IconShape=distinctive  AllPortsSameDT=off  OutDataTypeStr=boolean
  Sum : Outport
  CO : Outport  Port=2
  wires:
  B/1 -> B-Modifier/1
  Subtract/1 -> B-Modifier/2
  CI&&A^B/1 -> CO||/1
  A&&B/1 -> CO||/2  "AND"
  CO||/1 -> CO/1
  B-Modifier/1 -> A&&B/2, A^B/2  "B_M"
  CI/1 -> CI&&A^B/2, SUM/2
  A^B/1 -> CI&&A^B/1, SUM/1  "XOR"
  A/1 -> A&&B/1, A^B/1
  SUM/1 -> Sum/1

== system ProgramCounter/PC/Subsystem12/Subsystem6 ==
  A : Inport
  B : Inport  Port=2
  Subtract : Inport  Port=3
  CI : Inport  Port=4
  A&&B : Logic  IconShape=distinctive  AllPortsSameDT=off  OutDataTypeStr=boolean
  A^B : Logic  Operator=XOR  IconShape=distinctive  AllPortsSameDT=off  OutDataTypeStr=boolean
  B-Modifier : Logic  Operator=XOR  IconShape=distinctive  AllPortsSameDT=off  OutDataTypeStr=boolean
  CI&&A^B : Logic  IconShape=distinctive  AllPortsSameDT=off  OutDataTypeStr=boolean
  CO|| : Logic  Operator=OR  IconShape=distinctive  AllPortsSameDT=off  OutDataTypeStr=boolean
  SUM : Logic  Operator=XOR  IconShape=distinctive  AllPortsSameDT=off  OutDataTypeStr=boolean
  Sum : Outport
  CO : Outport  Port=2
  wires:
  B/1 -> B-Modifier/1
  Subtract/1 -> B-Modifier/2
  CI&&A^B/1 -> CO||/1
  A&&B/1 -> CO||/2  "AND"
  CO||/1 -> CO/1
  B-Modifier/1 -> A&&B/2, A^B/2  "B_M"
  CI/1 -> CI&&A^B/2, SUM/2
  A^B/1 -> CI&&A^B/1, SUM/1  "XOR"
  A/1 -> A&&B/1, A^B/1
  SUM/1 -> Sum/1

== system ProgramCounter/PC/Subsystem12/Subsystem7 ==
  A : Inport
  B : Inport  Port=2
  Subtract : Inport  Port=3
  CI : Inport  Port=4
  A&&B : Logic  IconShape=distinctive  AllPortsSameDT=off  OutDataTypeStr=boolean
  A^B : Logic  Operator=XOR  IconShape=distinctive  AllPortsSameDT=off  OutDataTypeStr=boolean
  B-Modifier : Logic  Operator=XOR  IconShape=distinctive  AllPortsSameDT=off  OutDataTypeStr=boolean
  CI&&A^B : Logic  IconShape=distinctive  AllPortsSameDT=off  OutDataTypeStr=boolean
  CO|| : Logic  Operator=OR  IconShape=distinctive  AllPortsSameDT=off  OutDataTypeStr=boolean
  SUM : Logic  Operator=XOR  IconShape=distinctive  AllPortsSameDT=off  OutDataTypeStr=boolean
  Sum : Outport
  CO : Outport  Port=2
  wires:
  B/1 -> B-Modifier/1
  Subtract/1 -> B-Modifier/2
  CI&&A^B/1 -> CO||/1
  A&&B/1 -> CO||/2  "AND"
  CO||/1 -> CO/1
  B-Modifier/1 -> A&&B/2, A^B/2  "B_M"
  CI/1 -> CI&&A^B/2, SUM/2
  A^B/1 -> CI&&A^B/1, SUM/1  "XOR"
  A/1 -> A&&B/1, A^B/1
  SUM/1 -> Sum/1

== system ProgramCounter/PC/Subsystem12/Subsystem8 ==
  A : Inport
  B : Inport  Port=2
  Subtract : Inport  Port=3
  CI : Inport  Port=4
  A&&B : Logic  IconShape=distinctive  AllPortsSameDT=off  OutDataTypeStr=boolean
  A^B : Logic  Operator=XOR  IconShape=distinctive  AllPortsSameDT=off  OutDataTypeStr=boolean
  B-Modifier : Logic  Operator=XOR  IconShape=distinctive  AllPortsSameDT=off  OutDataTypeStr=boolean
  CI&&A^B : Logic  IconShape=distinctive  AllPortsSameDT=off  OutDataTypeStr=boolean
  CO|| : Logic  Operator=OR  IconShape=distinctive  AllPortsSameDT=off  OutDataTypeStr=boolean
  SUM : Logic  Operator=XOR  IconShape=distinctive  AllPortsSameDT=off  OutDataTypeStr=boolean
  Sum : Outport
  CO : Outport  Port=2
  wires:
  B/1 -> B-Modifier/1
  Subtract/1 -> B-Modifier/2
  CI&&A^B/1 -> CO||/1
  A&&B/1 -> CO||/2  "AND"
  CO||/1 -> CO/1
  B-Modifier/1 -> A&&B/2, A^B/2  "B_M"
  CI/1 -> CI&&A^B/2, SUM/2
  A^B/1 -> CI&&A^B/1, SUM/1  "XOR"
  A/1 -> A&&B/1, A^B/1
  SUM/1 -> Sum/1

== system ProgramCounter/PC/Subsystem12/Subsystem9 ==
  A : Inport
  B : Inport  Port=2
  Subtract : Inport  Port=3
  CI : Inport  Port=4
  A&&B : Logic  IconShape=distinctive  AllPortsSameDT=off  OutDataTypeStr=boolean
  A^B : Logic  Operator=XOR  IconShape=distinctive  AllPortsSameDT=off  OutDataTypeStr=boolean
  B-Modifier : Logic  Operator=XOR  IconShape=distinctive  AllPortsSameDT=off  OutDataTypeStr=boolean
  CI&&A^B : Logic  IconShape=distinctive  AllPortsSameDT=off  OutDataTypeStr=boolean
  CO|| : Logic  Operator=OR  IconShape=distinctive  AllPortsSameDT=off  OutDataTypeStr=boolean
  SUM : Logic  Operator=XOR  IconShape=distinctive  AllPortsSameDT=off  OutDataTypeStr=boolean
  Sum : Outport
  CO : Outport  Port=2
  wires:
  B/1 -> B-Modifier/1
  Subtract/1 -> B-Modifier/2
  CI&&A^B/1 -> CO||/1
  A&&B/1 -> CO||/2  "AND"
  CO||/1 -> CO/1
  B-Modifier/1 -> A&&B/2, A^B/2  "B_M"
  CI/1 -> CI&&A^B/2, SUM/2
  A^B/1 -> CI&&A^B/1, SUM/1  "XOR"
  A/1 -> A&&B/1, A^B/1
  SUM/1 -> Sum/1
